simulink model "ODE2"  (R2018a)
settings: Solver=VariableStepAuto  StartTime=0.0  StopTime=40  RelTol=1e-3
settings Model: Creator=Abhishek Srivastava  LastModifiedBy=Abhishek Srivastava

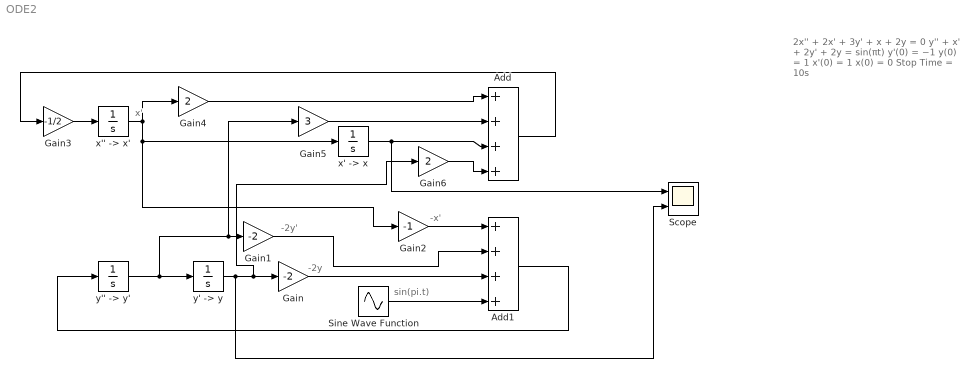
== system ODE2 ==
  note: -x'
  note: sin(pi.t)
  note: x'
  note: -2y
  note: -2y'
  note: 2x'' + 2x' + 3y' + x + 2y = 0
      | y'' + x' + 2y' + 2y = sin(πt)
      |
      | y'(0) = −1
      | y(0) = 1
      | x'(0) = 1
      | x(0) = 0
      |
      | Stop Time = 10s
  Add : Sum  Inputs=4
  Add1 : Sum  Inputs=4
  Gain : Gain  Gain=-2
  Gain1 : Gain  Gain=-2
  Gain2 : Gain  Gain=-1
  Gain3 : Gain  Gain=-1/2
  Gain4 : Gain  Gain=2
  Gain5 : Gain  Gain=3
  Gain6 : Gain  Gain=2
  Scope : Scope  NumInputPorts=2
  Sine Wave Function : Sin  Frequency=3.14  SampleTime=0
  "x' -> x" : Integrator
  "x'' -> x'" : Integrator  InitialCondition=1
  "y' -> y" : Integrator  InitialCondition=1
  "y'' -> y'" : Integrator  InitialCondition=-1
  wires:
  "y' -> y"/1 -> Scope/2, Gain6/1, Gain/1
  "y'' -> y'"/1 -> Gain5/1, Gain1/1, "y' -> y"/1
  Sine Wave Function/1 -> Add1/4
  Gain/1 -> Add1/3
  Gain1/1 -> Add1/2
  "x'' -> x'"/1 -> Gain4/1, Gain2/1, "x' -> x"/1
  Add/1 -> Gain3/1
  Add1/1 -> "y'' -> y'"/1
  Gain2/1 -> Add1/1
  Gain3/1 -> "x'' -> x'"/1
  Gain4/1 -> Add/1
  Gain5/1 -> Add/2
  "x' -> x"/1 -> Scope/1, Add/3
  Gain6/1 -> Add/4
